simulink model "mr_cpm_test1"  (R2014b)
settings: Solver=ode45  StartTime=0.0  StopTime=10.0  RelTol=1e-3
libraries: commdigbbndcpm2 x1, commrandsrc2 x1
settings Model: Creator=joel2  LastModifiedBy=joel2

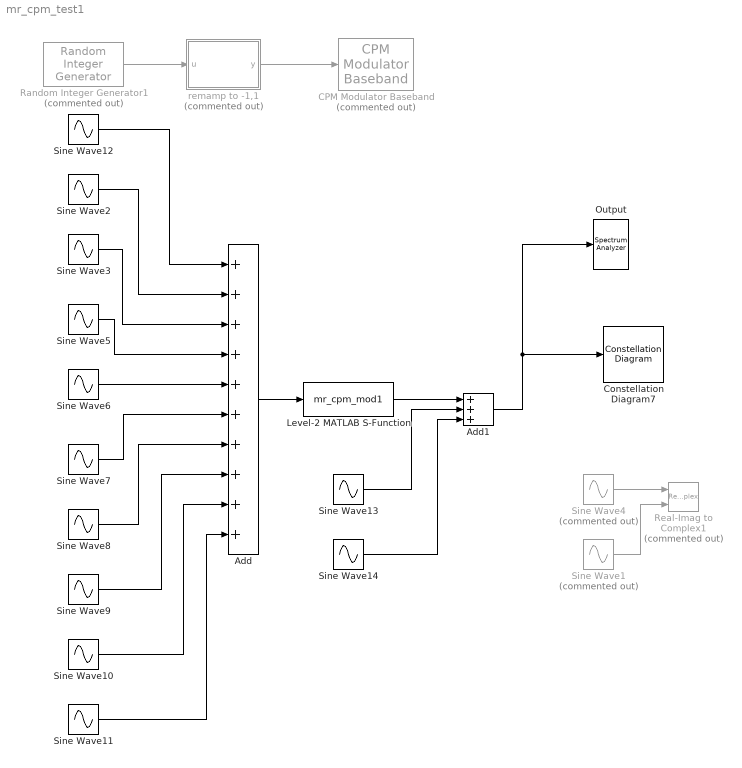
== system mr_cpm_test1 ==
  Add : Sum  Inputs=++++++++++
  Add1 : Sum  Inputs=+++
  CPM Modulator Baseband : commdigbbndcpm2/CPM Modulator Baseband  Commented=on  Mnum=4  inputType=Integer  mappingType=Binary  modIdx=0.5  pulseShape=Rectangular  BT=0.3  mainLobePulseLength=1  rollOff=0.2  pulseLength=1  preHistory=1  phaseOffset=0  samplesPerSymbol=8  RateOptions=Enforce single-rate processing  outDataType=double
  Constellation Diagram7 : ConstellationDiagram
  Level-2 MATLAB S-Function : M-S-Function  FunctionName=mr_cpm_mod1
  Output : SpectrumAnalyzer
  Random Integer Generator1 : commrandsrc2/Random Integer Generator  Commented=on  mul=2  seed=42  Ts=1/(10000)  frameBased=off  sampPerFrame=1024  orient=off  outDataType=double
  Real-Imag to Complex1 : RealImagToComplex  Commented=on
  Sine Wave1 : Sin  Commented=on  Frequency=12.801*2*pi*1000  Phase=-pi/2  SampleTime=1/128000
  Sine Wave10 : Sin  Amplitude=0.1  Frequency=98*2*pi  SampleTime=1/128000
  Sine Wave11 : Sin  Amplitude=0.1  Frequency=99*2*pi  SampleTime=1/128000
  Sine Wave12 : Sin  Amplitude=0.1  Frequency=100*2*pi  SampleTime=1/128000
  Sine Wave13 : Sin  Frequency=10*2*pi  SampleTime=1/128000
  Sine Wave14 : Sin  Frequency=20*2*pi  SampleTime=1/128000
  Sine Wave2 : Sin  Amplitude=0.1  Frequency=91*2*pi  SampleTime=1/128000
  Sine Wave3 : Sin  Amplitude=0.1  Frequency=92*2*pi  SampleTime=1/128000
  Sine Wave4 : Sin  Commented=on  Frequency=12.801*2*pi*1000  SampleTime=1/128000
  Sine Wave5 : Sin  Amplitude=0.1  Frequency=93*2*pi  SampleTime=1/128000
  Sine Wave6 : Sin  Amplitude=0.1  Frequency=94*2*pi  SampleTime=1/128000
  Sine Wave7 : Sin  Amplitude=0.1  Frequency=95*2*pi  SampleTime=1/128000
  Sine Wave8 : Sin  Amplitude=0.1  Frequency=96*2*pi  SampleTime=1/128000
  Sine Wave9 : Sin  Amplitude=0.1  Frequency=97*2*pi  SampleTime=1/128000
  remamp to -1,1 : MATLAB Function  Commented=on  TreatAsAtomicUnit=on
  wires:
  Sine Wave4/1 -> Real-Imag to Complex1/1
  Sine Wave1/1 -> Real-Imag to Complex1/2
  Random Integer Generator1/1 -> remamp to -1,1/1(u)
  remamp to -1,1/1(y) -> CPM Modulator Baseband/1
  Sine Wave12/1 -> Add/1
  Sine Wave2/1 -> Add/2
  Sine Wave3/1 -> Add/3
  Sine Wave5/1 -> Add/4
  Sine Wave6/1 -> Add/5
  Sine Wave7/1 -> Add/6
  Sine Wave8/1 -> Add/7
  Sine Wave9/1 -> Add/8
  Sine Wave10/1 -> Add/9
  Sine Wave11/1 -> Add/10
  Add/1 -> Level-2 MATLAB S-Function/1
  Level-2 MATLAB S-Function/1 -> Add1/1
  Sine Wave13/1 -> Add1/2
  Add1/1 -> Constellation Diagram7/1, Output/1
  Sine Wave14/1 -> Add1/3

== matlab function mr_cpm_test1/remamp to -1,1 ==
  data: u input; y output
function y = fcn(u)
%#codegen

y = (u*2)-1;
